simulink model "ANC_try1"  (R2020a)
settings: Solver=ode45  StartTime=0.0  StopTime=inf  RelTol=1e-3  EnableMultiTasking=on
libraries: dspvision x1, dspadpt3 x1, dspsrcs4 x1, dspobslib x1
settings Model: Creator=Aalim  LastModifiedBy=yjind
settings DataIOCC: LimitDataPoints=on  SaveFormat=Array  ReturnWorkspaceOutputs=off
settings OptimizationCC: ExpressionDepthLimit=2147483647  LifeSpan=inf
settings DebuggingCC: UnderspecifiedInitializationDetection=Classic  MergeDetectMultiDrivingBlocksExec=none  SolverPrmCheckMsg=warning  StateNameClashWarn=warning  SFUnexpectedBacktrackingDiag=warning  SFNoUnconditionalDefaultTransitionDiag=warning  SFExecutionAtInitializationDiag=none  ArithmeticOperatorsInVariantConditions=warning
settings HardwareCC: ProdBitPerPointer=32  ProdBitPerSizeT=32  ProdBitPerPtrDiffT=32  ProdLargestAtomicFloat=None  ProdIntDivRoundTo=Undefined  ProdEndianess=Unspecified  ProdWordSize=32  ProdHWDeviceType=32-bit Generic
settings ModelReferenceCC: PropagateSignalLabelsOutOfModel=off
settings SFSimCC: SimUseLocalCustomCode=off  CustomCodeUndefinedFunction=UseInterfaceOnly
settings RTWCC: RTWUseLocalCustomCode=off
settings CodeAppCC: StateflowObjectComments=on
settings GRTTargetCC: TargetLangStandard=C89/C90 (ANSI)
settings ConfigComp: CovMetricSettings=dw  CovHtmlReporting=on  CovSaveCumulativeToWorkspaceVar=on  CovSaveSingleToWorkspaceVar=on  CovExternalEMLEnable=off

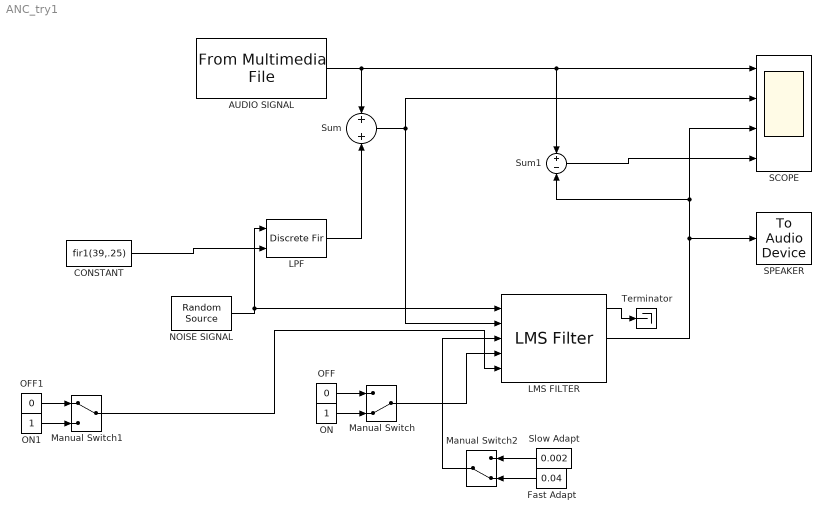
== system ANC_try1 ==
  AUDIO SIGNAL : dspvision/From Multimedia File  inputFilename=C:\Program Files\Polyspace\R2020a\toolbox\dsp\dsp\dspafxf_8000.wav  readRange=[1 Inf]  loop=on  numPlays=inf  outputStreams=Audio only  videoDataType=single  audioDataType=single  inheritSampleTime=on  userDefinedSampleTime=1/30  noAudioOutput=off  isIntensityVideo=off  fourcc=RGB  colorVideoFormat=Separate color signals  outputEOF=off  dataOrg=Column-major  audioFrameSize=32  computeAudioFrameSize=off  outSamplingMode=Sample based
  CONSTANT : Constant  Value=fir1(39,.25)  OutDataTypeStr=Inherit: Inherit via back propagation
  Fast Adapt : Constant  Value=0.04  OutDataTypeStr=Inherit: Inherit via back propagation
  LMS FILTER : dspadpt3/LMS Filter  Algo=Normalized LMS  L=40  stepflag=Input port  mu=0.0008  leakage=1.0  ic=0  Adapt=on  resetflag=Non-zero sample  weights=on  addnparflag=off  roundingMode=Floor  overflowMode=off  secondCoeffMode=Binary point scaling  secondCoeffWordLength=2  secondCoeffFracLength=15  prodOutput2Mode=Binary point scaling  prodOutput2FracLength=20  prodOutput3Mode=Binary point scaling  prodOutput3FracLength=20  prodOutput4Mode=Binary point scaling  prodOutput4FracLength=20  quotientMode=Binary point scaling  quotientFracLength=20  accum2Mode=Binary point scaling  accum2FracLength=20
      settings: SourceProductBaseCode=DS
  LPF : DiscreteFir  CoefSource=Input port  InputProcessing=Columns as channels (frame based)  AccumDataTypeStr=Inherit: Same as product output  OutDataTypeStr=Inherit: Same as input
      settings: InputPortMap=u0,u1
  Manual Switch : ManualSwitch  CurrentSetting=0
  Manual Switch1 : ManualSwitch
  Manual Switch2 : ManualSwitch  CurrentSetting=0
  NOISE SIGNAL : dspsrcs4/Random Source  SrcType=Gaussian  NormMethod=Sum of uniform values  CltLength=5  MinVal=0  MaxVal=1  MeanVal=0  VarVal=1  RepMode=Specify seed  rawSeed=[23341]  IsInherit=off  SampMode=Discrete  SampTime=1/8000  SampFrame=32  DataType=Single  OutComplex=Real  OutputFrames=on
  OFF : Constant  Value=0
  OFF1 : Constant  Value=0
  ON : Constant
  ON1 : Constant
  SCOPE : Scope  NumInputPorts=4
  SPEAKER : dspobslib/To Audio Device  deviceName=Primary Sound Driver  inheritSampleRate=on  sampleRate=44100  deviceDatatype=Determine from input data type  autoBufferSize=on  bufferSize=4096  queueDuration=1.0  defaultOutputChannelMapping=on  outputChannelMapping=1:2  outputNumUnderrunSamples=off
      settings: SourceProductBaseCode=DS
  Slow Adapt : Constant  Value=0.002  OutDataTypeStr=Inherit: Inherit via back propagation
  Sum : Sum  Inputs=+|+
  Sum1 : Sum  Inputs=+|-
  Terminator : Terminator
  wires:
  LMS FILTER/1 -> Terminator/1
  LMS FILTER/2 -> SCOPE/3, Sum1/2, SPEAKER/1
  LPF/1 -> Sum/2
  OFF/1 -> Manual Switch/1
  ON/1 -> Manual Switch/2
  Manual Switch/1 -> LMS FILTER/4
  AUDIO SIGNAL/1 -> SCOPE/1, Sum1/1, Sum/1
  Sum/1 -> LMS FILTER/2, SCOPE/2
  NOISE SIGNAL/1 -> LPF/1, LMS FILTER/1
  Manual Switch1/1 -> LMS FILTER/5
  ON1/1 -> Manual Switch1/2
  OFF1/1 -> Manual Switch1/1
  CONSTANT/1 -> LPF/2
  Fast Adapt/1 -> Manual Switch2/2
  Slow Adapt/1 -> Manual Switch2/1
  Manual Switch2/1 -> LMS FILTER/3
  Sum1/1 -> SCOPE/4
